simulink model "closedloop"  (R2025b)
settings: Solver=ode3  StartTime=0.0  StopTime=1.5  FixedStep=1e-5  MaxStep=1e-4  RelTol=1e-3
values from neighbouring files (symbols this model uses):
  C = 470*10^-6    (= 0.00047)    [plotting.m]    (also in robusnost_grafici.m)
  L = 15.91*10^-3    (= 0.01591)    [plotting.m]    (also in robusnost_grafici.m = 0.012728)
  poremecaj = 0.8    [plotting.m]    (also in robusnost_grafici.m)
  R = 52    [plotting.m]    (also in robusnost_grafici.m)
  sig2 = (0.02*x2e)^2    (= 0.2025)    [plotting.m]    (also in robusnost_grafici.m = 0)
  x2e = Vc    (= -22.5)    [plotting.m]    (also in robusnost_grafici.m)
undefined symbols (not defined in the file or in its folder): den, num
settings Model: Creator=Administrator  LastModifiedBy=User

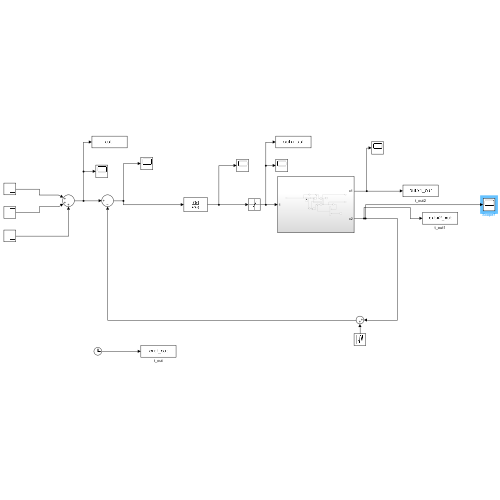
[thumbnail: Simulink's stored preview of the top-level diagram]
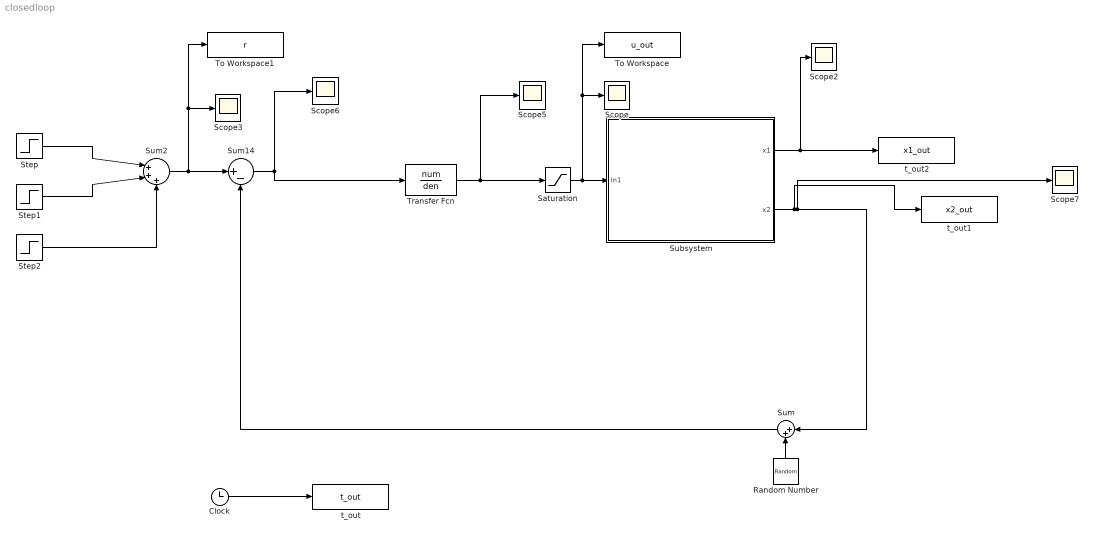
== system closedloop ==
  Clock : Clock
  Random Number : RandomNumber  Variance=sig2  SampleTime=1e-5
  Saturation : Saturate  UpperLimit=1  LowerLimit=0
  Scope{,2..3,5..7} (6 alike) : Scope
      Scope settings: ActiveDisplayYMinimum=0.635540716527341  ActiveDisplayYMaximum=0.6984625525624738
      Scope2 settings: ActiveDisplayYMinimum=-48122.298108466144  ActiveDisplayYMaximum=89272.874926725228  DataLoggingVariableName=ScopeData2
      Scope3 settings: ActiveDisplayYMinimum=-22.1336544866135  ActiveDisplayYMaximum=2.7956236481533843  DataLoggingVariableName=ScopeData3
      Scope5 settings: ActiveDisplayYMinimum=-34.759715926741777  ActiveDisplayYMaximum=3.8621906585268628  DataLoggingVariableName=ScopeData5
      Scope6 settings: ActiveDisplayYMinimum=-83.976264055231624  ActiveDisplayYMaximum=45.322775175454908  DataLoggingVariableName=ScopeData6
      Scope7 settings: ActiveDisplayYMinimum=-32.16394623834028  ActiveDisplayYMaximum=-13.816916408919962  DataLoggingVariableName=ScopeData7
  Step : Step  Time=0  After=x2e  SampleTime=0
  Step1 : Step  Time=0.5  After=5  SampleTime=0
  Step2 : Step  After=-5  SampleTime=0
  Subsystem : Subsystem
  Sum : Sum  Inputs=|++
  Sum14 : Sum  Inputs=|+-
  Sum2 : Sum  Inputs=|+++
  To Workspace : ToWorkspace  VariableName=u_out  SampleTime=-1
  To Workspace1 : ToWorkspace  VariableName=r  SampleTime=-1
  Transfer Fcn : TransferFcn  Numerator=num  Denominator=den
  t_out : ToWorkspace  VariableName=t_out  SampleTime=-1
  t_out1 : ToWorkspace  VariableName=x2_out  SampleTime=-1
  t_out2 : ToWorkspace  VariableName=x1_out  SampleTime=-1
  wires:
  Subsystem/1(x1) -> Scope2/1, t_out2/1
  Sum2/1 -> Sum14/1, Scope3/1, To Workspace1/1
  Saturation/1 -> To Workspace/1, Scope/1, Subsystem/1(In1)
  Clock/1 -> t_out/1
  Sum14/1 -> Scope6/1, Transfer Fcn/1
  Transfer Fcn/1 -> Saturation/1, Scope5/1
  Subsystem/2(x2) -> t_out1/1, Sum/1, Scope7/1
  Sum/1 -> Sum14/2
  Random Number/1 -> Sum/2
  Step/1 -> Sum2/1
  Step1/1 -> Sum2/2
  Step2/1 -> Sum2/3

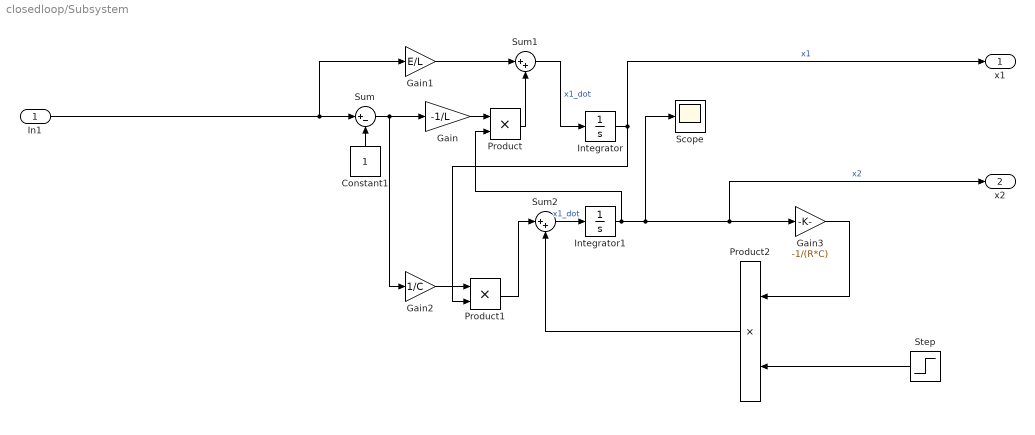
== system closedloop/Subsystem ==
  In1 : Inport
  Constant1 : Constant
  Gain : Gain  Gain=-1/L
  Gain1 : Gain  Gain=E/L
  Gain2 : Gain  Gain=1/C
  Gain3 : Gain  Gain=-1/(R*C)
  Integrator : Integrator
  Integrator1 : Integrator
  Product : Product
  Product1 : Product
  Product2 : Product
  Scope : Scope
      settings: ActiveDisplayYMinimum=-21.097117742306263  ActiveDisplayYMaximum=-19.897993351884285  DataLoggingVariableName=ScopeData8
  Step : Step  Time=1.3  Before=1  After=1/poremecaj  SampleTime=0
  Sum : Sum  Inputs=|+-
  Sum1 : Sum  Inputs=|++
  Sum2 : Sum  Inputs=|++
  x1 : Outport
  x2 : Outport  Port=2
  wires:
  Gain/1 -> Product/1
  In1/1 -> Gain1/1, Sum/1
  Sum1/1 -> Integrator/1  "x1_dot"
  Gain1/1 -> Sum1/1
  Sum/1 -> Gain2/1, Gain/1
  Constant1/1 -> Sum/2
  Gain2/1 -> Product1/1
  Product/1 -> Sum1/2
  Integrator1/1 -> x2/1, Gain3/1, Scope/1, Product/2  "x2"
  Product1/1 -> Sum2/1
  Integrator/1 -> x1/1, Product1/2  "x1"
  Sum2/1 -> Integrator1/1  "x1_dot"
  Product2/1 -> Sum2/2
  Gain3/1 -> Product2/1
  Step/1 -> Product2/2
